simulink model "Vehicle_Acceleration"  (R2013a)
settings: Solver=ode45  StartTime=0.0  StopTime=10.0  RelTol=1e-3
libraries: simulink x18
settings Model: Creator=KAI - PC  LastModifiedBy=Admin
settings DataIOCC: SignalLoggingSaveFormat=ModelDataLogs
settings OptimizationCC: ExpressionDepthLimit=2147483647
settings DebuggingCC: FcnCallInpInsideContextMsg=EnableAllAsWarning

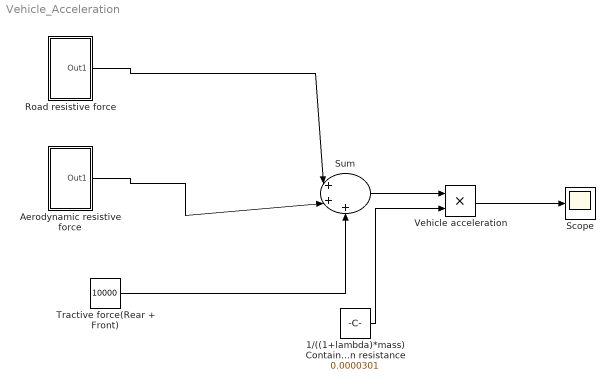
== system Vehicle_Acceleration ==
  1/((1+lambda)*mass) Contains acceleration resistance : Constant  Value=0.0000301
  Aerodynamic resistive force : Subsystem
  Road resistive force : Subsystem
  Scope : Scope
  Sum : Sum  Inputs=|+++
  Tractive force(Rear + Front) : Constant  Value=10000
  Vehicle acceleration : Product  RndMeth=Zero
  wires:
  Road resistive force/1(Out1) -> Sum/1
  Aerodynamic resistive force/1(Out1) -> Sum/2
  Tractive force(Rear + Front)/1 -> Sum/3
  Sum/1 -> Vehicle acceleration/1
  1/((1+lambda)*mass) Contains acceleration resistance/1 -> Vehicle acceleration/2
  Vehicle acceleration/1 -> Scope/1

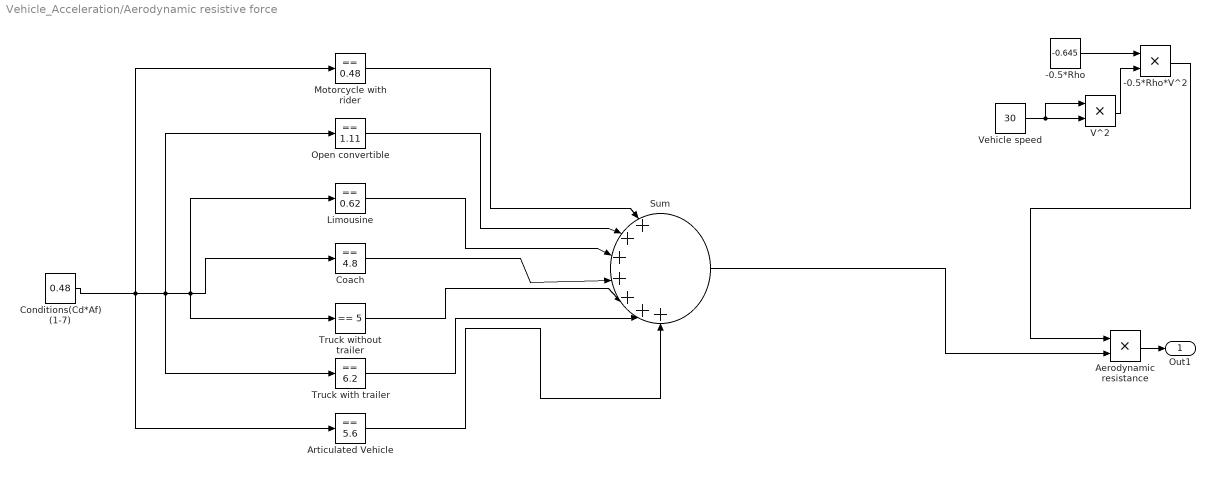
== system Vehicle_Acceleration/Aerodynamic resistive force ==
  -0.5*Rho : Constant  Value=-0.645
  -0.5*Rho*V^2 : Product  RndMeth=Zero
  Aerodynamic resistance : Product  RndMeth=Zero
  Articulated Vehicle : simulink/Logic and Bit Operations/Compare To Constant  relop===  const=5.6  OutDataTypeStr=uint8
  Coach : simulink/Logic and Bit Operations/Compare To Constant  relop===  const=4.8  OutDataTypeStr=uint8
  Conditions(Cd*Af) (1-7) : Constant  Value=0.48
  Limousine : simulink/Logic and Bit Operations/Compare To Constant  relop===  const=0.62  OutDataTypeStr=uint8
  "Motorcycle with rider " : simulink/Logic and Bit Operations/Compare To Constant  relop===  const=0.48  OutDataTypeStr=uint8
  Open convertible : simulink/Logic and Bit Operations/Compare To Constant  relop===  const=1.11  OutDataTypeStr=uint8
  Sum : Sum  Inputs=|+++++++
  Truck with trailer : simulink/Logic and Bit Operations/Compare To Constant  relop===  const=6.2  OutDataTypeStr=uint8
  Truck without trailer : simulink/Logic and Bit Operations/Compare To Constant  relop===  const=5  OutDataTypeStr=uint8
  V^2 : Product  RndMeth=Zero
  Vehicle speed : Constant  Value=30
  Out1 : Outport
  wires:
  Vehicle speed/1 -> V^2/2, V^2/1
  "Motorcycle with rider "/1 -> Sum/1
  Open convertible/1 -> Sum/2
  Limousine/1 -> Sum/3
  Coach/1 -> Sum/4
  Articulated Vehicle/1 -> Sum/7
  Truck with trailer/1 -> Sum/6
  Truck without trailer/1 -> Sum/5
  Conditions(Cd*Af) (1-7)/1 -> Coach/1, Truck without trailer/1, Limousine/1, Truck with trailer/1, Open convertible/1, Articulated Vehicle/1, "Motorcycle with rider "/1
  -0.5*Rho/1 -> -0.5*Rho*V^2/1
  V^2/1 -> -0.5*Rho*V^2/2
  -0.5*Rho*V^2/1 -> Aerodynamic resistance/1
  Aerodynamic resistance/1 -> Out1/1
  Sum/1 -> Aerodynamic resistance/2

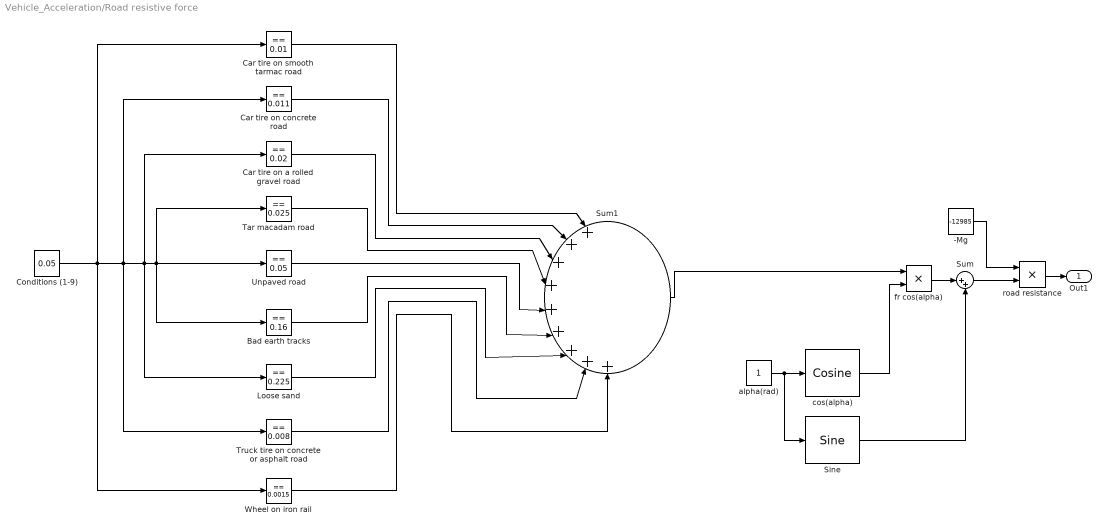
== system Vehicle_Acceleration/Road resistive force ==
  "-Mg " : Constant  Value=-12985
  Bad earth tracks : simulink/Logic and Bit Operations/Compare To Constant  relop===  const=0.16  OutDataTypeStr=uint8
  "Car tire on a rolled gravel road " : simulink/Logic and Bit Operations/Compare To Constant  relop===  const=0.02  OutDataTypeStr=uint8
  Car tire on concrete road : simulink/Logic and Bit Operations/Compare To Constant  relop===  const=0.011  OutDataTypeStr=uint8
  "Car tire on smooth tarmac road " : simulink/Logic and Bit Operations/Compare To Constant  relop===  const=0.01  OutDataTypeStr=uint8
  Conditions (1-9) : Constant  Value=0.05
  Loose sand : simulink/Logic and Bit Operations/Compare To Constant  relop===  const=0.225  OutDataTypeStr=uint8
  Sine : simulink/Lookup Tables/Sine  Formula=sin(2*pi*u)  NumDataPoints=(2^5)+1  OutputWordLength=16
  Sum : Sum  Inputs=|++
  Sum1 : Sum  Inputs=|+++++++++
  Tar macadam road : simulink/Logic and Bit Operations/Compare To Constant  relop===  const=0.025  OutDataTypeStr=uint8
  Truck tire on concrete or asphalt road : simulink/Logic and Bit Operations/Compare To Constant  relop===  const=0.008  OutDataTypeStr=uint8
  Unpaved road : simulink/Logic and Bit Operations/Compare To Constant  relop===  const=0.05  OutDataTypeStr=uint8
  Wheel on iron rail : simulink/Logic and Bit Operations/Compare To Constant  relop===  const=0.0015  OutDataTypeStr=uint8
  alpha(rad) : Constant
  cos(alpha) : simulink/Lookup Tables/Cosine  Formula=cos(2*pi*u)  NumDataPoints=(2^5)+1  OutputWordLength=16
  fr cos(alpha) : Product  RndMeth=Zero
  road resistance : Product  RndMeth=Zero
  Out1 : Outport
  wires:
  Conditions (1-9)/1 -> "Car tire on smooth tarmac road "/1, Car tire on concrete road/1, "Car tire on a rolled gravel road "/1, Unpaved road/1, Tar macadam road/1, Bad earth tracks/1, Loose sand/1, Truck tire on concrete or asphalt road/1, Wheel on iron rail/1
  Unpaved road/1 -> Sum1/5
  Bad earth tracks/1 -> Sum1/6
  Loose sand/1 -> Sum1/7
  Truck tire on concrete or asphalt road/1 -> Sum1/8
  Wheel on iron rail/1 -> Sum1/9
  Tar macadam road/1 -> Sum1/4
  "Car tire on a rolled gravel road "/1 -> Sum1/3
  Car tire on concrete road/1 -> Sum1/2
  "Car tire on smooth tarmac road "/1 -> Sum1/1
  cos(alpha)/1 -> fr cos(alpha)/2
  Sum1/1 -> fr cos(alpha)/1
  alpha(rad)/1 -> cos(alpha)/1, Sine/1
  fr cos(alpha)/1 -> Sum/1
  Sine/1 -> Sum/2
  Sum/1 -> road resistance/2
  "-Mg "/1 -> road resistance/1
  road resistance/1 -> Out1/1
